simulink model "L0301"  (R2022b)
settings: Solver=VariableStepAuto  StartTime=0.0  StopTime=10.0  RelTol=1e-3
libraries: simulink x4
settings Model: Creator=Andrey  LastModifiedBy=Andrey

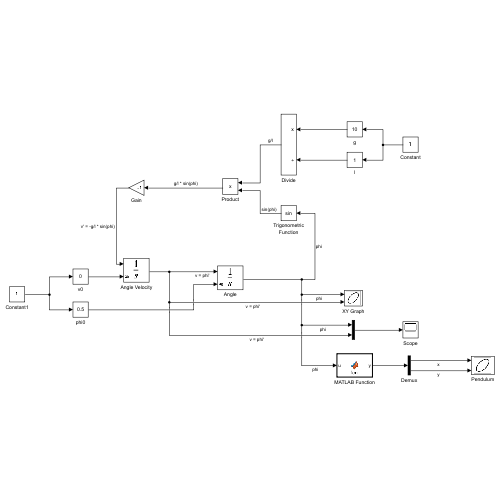
[thumbnail: Simulink's stored preview of the top-level diagram]
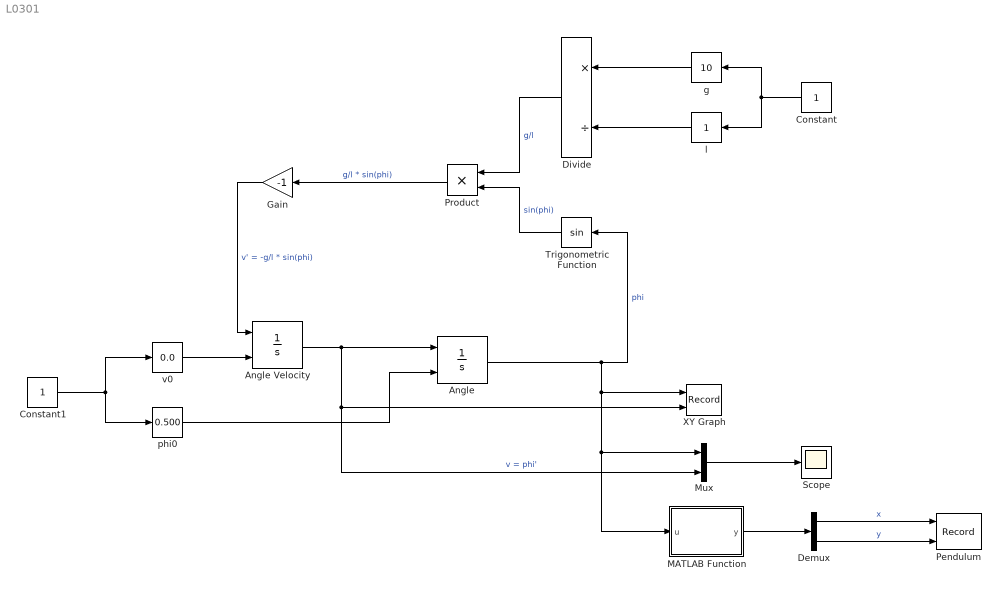
== system L0301 ==
  Angle : Integrator  InitialConditionSource=external
  Angle Velocity : Integrator  InitialConditionSource=external
  Constant : Constant
  Constant1 : Constant
  Demux : Demux  Outputs=2
  Divide : Product  Inputs=*/
  Gain : Gain  Gain=-1
  MATLAB Function : MATLAB Function  TreatAsAtomicUnit=on
  Mux : Mux  Inputs=2
  Pendulum : Record  FileSettingsInternal="{\"entries\":[{\"content\":{\"excelSettings\":{\"content\":{},\"type\":\"Streamout.ExcelSettings\"}},\"type\":\"Streamout.FileSettingStorage\",\"uuid\":\"d83f7bc0-736a-4460-a03a-272b2ec99242\"}],\"packageUris\":[\"http://schema.mathworks.com/mf0/streamout_blocks/R2020a\"],\"version\":\"1.0\"}"  Layout=[1 1]  SignalsInternal="{\"entries\":[{\"content\":{\"signals\":[{\"content\":{\"blockPath\":[\"L0301/Pendulum\"],\"channel\":[],\"dimensions\":[1,1],\"domain\":\"L0301/Pendulum\",\"lineColor\":\"#a2142f\",\"plots\":[1],\"port\":1,\"sid\":[\"\"],\"signalID\":302,\"signalName\":\"x\"},\"type\":\"RecordBlkView.Signal\",\"uuid\":\"357e23c5-d5a2-4d56-b6e5-249eec3b144e\"},{\"content\":{\"blockPath\":[\"L0301/Pendulum\"],\"channel\":[],\"dimensions\":[1,1],\"domain\":\"L0301/Pendulum\",\"lineColor\":\"#139fff\",\"plots\":[1],\"port\":2,\"sid\":[\"\"],\"signalID\":306,\"signalName\":\"y\"},\"type\":\"RecordBlkView.Signal\",\"uuid\":\"170b6974-ff03-4d60-8147-5eb95fbc5787\"}]},\"type\":\"RecordBlkView.InputSignals\",\"uuid\":\"d5dfb3d0-a3cd-45c8-bcae-a58686abcd4c\"}],\"packageUris\":[\"http://schema.mathworks.com/mf0/streamout_blocks/R2020a\"],\"version\":\"1.0\"}"  VisualizationBindings="{\"xyplotplugin\":{\"info\":[{\"series\":[{\"bindingParametersList\":[{\"parameter\":\"Y-Axis\",\"signalID\":306,\"signalName\":\"y\"},{\"parameter\":\"X-Axis\",\"signalID\":302,\"signalName\":\"x\"}],\"seriesID\":27802}],\"subplotID\":1}]}}"  CompatibilityTag=XY
  Product : Product
  Scope : Scope
  Trigonometric Function : Trigonometry
  XY Graph : Record  FileSettingsInternal="{\"entries\":[{\"content\":{\"excelSettings\":{\"content\":{},\"type\":\"Streamout.ExcelSettings\"}},\"type\":\"Streamout.FileSettingStorage\",\"uuid\":\"871bfbfd-5b56-4b8f-9c82-94ac53a41776\"}],\"packageUris\":[\"http://schema.mathworks.com/mf0/streamout_blocks/R2020a\"],\"version\":\"1.0\"}"  Layout=[1 1]  SignalsInternal="{\"entries\":[{\"content\":{\"signals\":[{\"content\":{\"blockPath\":[\"L0301/XY Graph\"],\"channel\":[],\"dimensions\":[1],\"domain\":\"L0301/XY Graph\",\"lineColor\":\"#0072bd\",\"plots\":[1],\"port\":1,\"sid\":[\"\"],\"signalID\":310,\"signalName\":\"phi\"},\"type\":\"RecordBlkView.Signal\",\"uuid\":\"37d274fa-b6d2-4492-b20f-881183a2afac\"},{\"content\":{\"blockPath\":[\"L0301/XY Graph\"],\"channel\":[],\"dimensions\":[1],\"domain\":\"L0301/XY Graph\",\"lineColor\":\"#d95319\",\"plots\":[1],\"port\":2,\"sid\":[\"\"],\"signalID\":314,\"signalName\":\"v = phi'\"},\"type\":\"RecordBlkView.Signal\",\"uuid\":\"fc989b2c-49a6-4b34-8bdb-15152256e8b2\"}]},\"type\":\"RecordBlkView.InputSignals\",\"uuid\":\"2a237a29-0bff-41e9-ada3-6e28788157d2\"}],\"packageUris\":[\"http://schema.mathworks.com/mf0/streamout_blocks/R2020a\"],\"version\":\"1.0\"}"  VisualizationBindings="{\"xyplotplugin\":{\"info\":[{\"series\":[{\"bindingParametersList\":[{\"parameter\":\"Y-Axis\",\"signalID\":314,\"signalName\":\"v = phi'\"},{\"parameter\":\"X-Axis\",\"signalID\":310,\"signalName\":\"phi\"}],\"seriesID\":50716}],\"subplotID\":1}]}}"  CompatibilityTag=XY
  g : simulink/Math Operations/Slider Gain  gain=10  low=0  high=10
  l : simulink/Math Operations/Slider Gain  gain=1  low=0  high=2
  phi0 : simulink/Math Operations/Slider Gain  gain=0.500  low=0  high=2
  v0 : simulink/Math Operations/Slider Gain  gain=0.0  low=0  high=2
  wires:
  Angle Velocity/1 -> Angle/1, Mux/2, XY Graph/2  "v = phi'"
  Angle/1 -> Trigonometric Function/1, MATLAB Function/1(u), Mux/1, XY Graph/1  "phi"
  Constant/1 -> l/1, g/1
  g/1 -> Divide/1
  l/1 -> Divide/2
  Trigonometric Function/1 -> Product/2  "sin(phi)"
  Divide/1 -> Product/1  "g/l"
  Product/1 -> Gain/1  "g/l * sin(phi)"
  Gain/1 -> Angle Velocity/1  "v' = -g/l * sin(phi)"
  Mux/1 -> Scope/1
  v0/1 -> Angle Velocity/2
  phi0/1 -> Angle/2
  Constant1/1 -> phi0/1, v0/1
  MATLAB Function/1(y) -> Demux/1
  Demux/1 -> Pendulum/1  "x"
  Demux/2 -> Pendulum/2  "y"

== matlab function L0301/MATLAB Function ==
  data: u input; y output
function y  = fcn(u)
%#codegen

y = [sin(u),-cos(u)]';
